simulink model "ScpAp_SpeedSupervision"  (R2025b)
settings: Solver=FixedStepDiscrete  StartTime=0.0  StopTime=10.0  FixedStep=0.01  RelTol=1e-3
model workspace (MAT data in the model file):
  K_Pred = Simulink.Parameter
  K_Pred.Value = 0.003
  K_Pred.Complexity = 'real'
  K_Pred.Dimensions = [1 1]
  K_Pred.DataType = 'auto'
  TH_Hystersis = Simulink.Parameter
  TH_Hystersis.Value = 3
  TH_Hystersis.Complexity = 'real'
  TH_Hystersis.Dimensions = [1 1]
  TH_Hystersis.DataType = 'auto'
  TH_Mon_Accel_Diff = Simulink.Parameter
  TH_Mon_Accel_Diff.Value = 2
  TH_Mon_Accel_Diff.Complexity = 'real'
  TH_Mon_Accel_Diff.Dimensions = [1 1]
  TH_Mon_Accel_Diff.DataType = 'auto'
  TH_Mon_Speed_Diff = Simulink.Parameter
  TH_Mon_Speed_Diff.Value = 2
  TH_Mon_Speed_Diff.Complexity = 'real'
  TH_Mon_Speed_Diff.Dimensions = [1 1]
  TH_Mon_Speed_Diff.DataType = 'auto'
  TH_Pred_Margin = Simulink.Parameter
  TH_Pred_Margin.Value = 2
  TH_Pred_Margin.Complexity = 'real'
  TH_Pred_Margin.Dimensions = [1 1]
  TH_Pred_Margin.DataType = 'auto'
  TH_Speed_Limit_Margin = Simulink.Parameter
  TH_Speed_Limit_Margin.Value = 3
  TH_Speed_Limit_Margin.Complexity = 'real'
  TH_Speed_Limit_Margin.Dimensions = [1 1]
  TH_Speed_Limit_Margin.DataType = 'auto'
  Torque_Decel_Limit = Simulink.Parameter
  Torque_Decel_Limit.Value = 500
  Torque_Decel_Limit.Complexity = 'real'
  Torque_Decel_Limit.Dimensions = [1 1]
  Torque_Decel_Limit.DataType = 'auto'
  Torque_PreLimit = Simulink.Parameter
  Torque_PreLimit.Value = 600
  Torque_PreLimit.Complexity = 'real'
  Torque_PreLimit.Dimensions = [1 1]
  Torque_PreLimit.DataType = 'auto'
undefined symbols (not defined in the file): SafetyMode_L2p_IDT, WhlSpd_Max
settings Model: DataDictionary=EgasPOC.sldd  Creator=IAST283  LastModifiedBy=IAST283
settings DataIOCC: SaveFormat=StructureWithTime
settings OptimizationCC: DefaultParameterBehavior=Inlined  EnhancedBackFolding=on  PassReuseOutputArgsAs=Individual arguments  ZeroExternalMemoryAtStartup=off  ZeroInternalMemoryAtStartup=off  OptimizeBlockOrder=speed  DifferentSizesBufferReuse=on  OptimizationCustomize=off  EfficientTunableParamExpr=on
settings DebuggingCC: ParameterTunabilityLossMsg=error
settings SFSimCC: MATLABDynamicMemAlloc=off
settings RTWCC: SystemTargetFile=autosar.tlc  GenCodeOnly=on  TemplateMakefile=ert_default_tmf  DataTypeReplacement=CDataTypesFixedWidth  Description=AUTOSAR
settings CodeAppCC: ForceParamTrailComments=on  IgnoreCustomStorageClasses=off  OperatorAnnotations=on  SimulinkDataObjDesc=on  SFDataObjDesc=on  InsertBlockDesc=on
settings STFCustomTargetCC: SystemTargetFile=autosar.tlc  TargetLangStandard=C99 (ISO)  MultiwordLength=256.0  ParMdlRefBuildCompliant=on  CompOptLevelCompliant=on  ConcurrentExecutionCompliant=off  IncludeMdlTerminateFcn=off  CombineOutputUpdateFcns=on  SuppressErrorStatus=on  ERTCustomFileBanners=on  SupportNonFinite=off  SupportComplex=off  SupportContinuousTime=off  SupportNonInlinedSFcns=off  RemoveResetFunc=on  MATLABClassNameForMDSCustomization=Simulink.SoftwareTarget.ERTCustomization  AutosarCompliant=on  GRTInterface=off  UseToolchainInfoCompliant=on  LookupTableObjectStructAxisOrder=2,1,3,4,...  LUTObjectStructOrderEvenSpacing=Size,Table,Breakpoints  AutosarMatrixIOAsArray=off  AutosarCompilerAbstraction=off  AutosarMaxShortNameLength=128.0  AutosarSchemaVersion=R20-11  DisableAUTOSARRoutinesHostLibrary=off
settings ERTTargetCC: ERTCustomFileTemplate=example_file_process.tlc  BooleanTrueId=TRUE  BooleanFalseId=FALSE  TargetLangStandard=C99 (ISO)  ConcurrentExecutionCompliant=off  IncludeMdlTerminateFcn=off  SuppressErrorStatus=on  SupportNonFinite=off  SupportComplex=off  ModelStepFunctionPrototypeControlCompliant=off  CPPClassGenCompliant=off  AutosarCompliant=on  LookupTableObjectStructAxisOrder=2,1,3,4,...  LUTObjectStructOrderEvenSpacing=Size,Table,Breakpoints

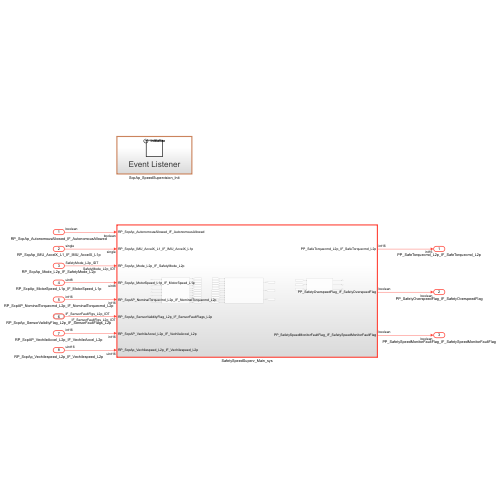
[thumbnail: Simulink's stored preview of the top-level diagram]
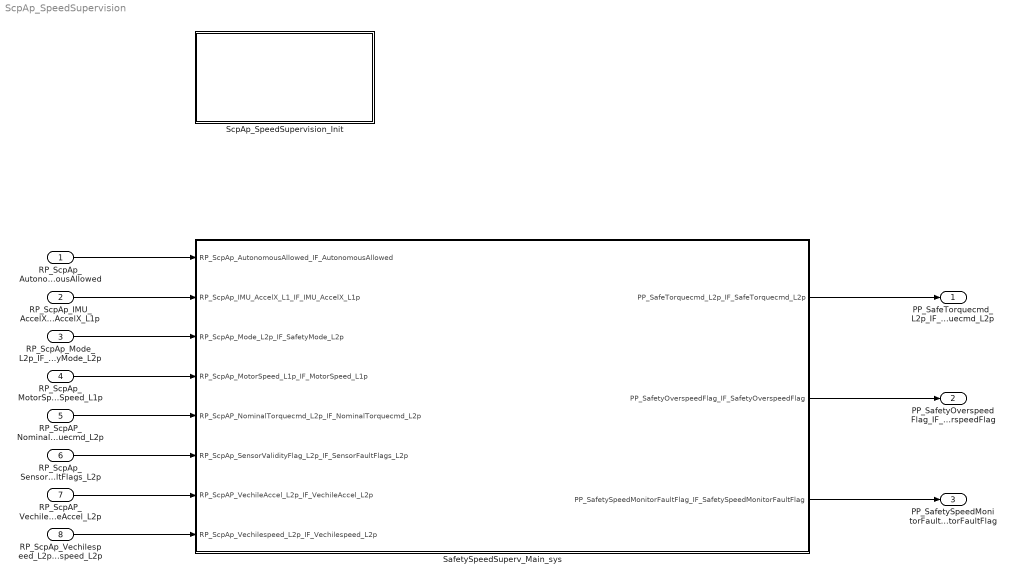
== system ScpAp_SpeedSupervision ==
  RP_ScpAp_AutonomousAllowed_IF_AutonomousAllowed : Inport  OutDataTypeStr=boolean  PortDimensions=1
  RP_ScpAp_IMU_AccelX_L1_IF_IMU_AccelX_L1p : Inport  Port=2  OutDataTypeStr=single  PortDimensions=1
  RP_ScpAp_Mode_L2p_IF_SafetyMode_L2p : Inport  Port=3  OutDataTypeStr=Enum: SafetyMode_L2p_IDT  PortDimensions=1
  RP_ScpAp_MotorSpeed_L1p_IF_MotorSpeed_L1p : Inport  Port=4  OutDataTypeStr=uint8  PortDimensions=1
  RP_ScpAP_NominalTorquecmd_L2p_IF_NominalTorquecmd_L2p : Inport  Port=5  OutDataTypeStr=int16  PortDimensions=1
  RP_ScpAp_SensorValidityFlag_L2p_IF_SensorFaultFlags_L2p : Inport  Port=6  OutDataTypeStr=Bus: IF_SensorFaultFlgs_L2p_IDT  PortDimensions=1  BusOutputAsStruct=on
  RP_ScpAP_VechileAccel_L2p_IF_VechileAccel_L2p : Inport  Port=7  OutDataTypeStr=int16  PortDimensions=1
  RP_ScpAp_Vechilespeed_L2p_IF_Vechilespeed_L2p : Inport  Port=8  OutDataTypeStr=uint16  PortDimensions=1
  SafetySpeedSuperv_Main_sys : Subsystem  TreatAsAtomicUnit=on  SystemSampleTime=0.01
  ScpAp_SpeedSupervision_Init : Subsystem
  PP_SafeTorquecmd_L2p_IF_SafeTorquecmd_L2p : Outport  OutDataTypeStr=int16  PortDimensions=1
  PP_SafetyOverspeedFlag_IF_SafetyOverspeedFlag : Outport  Port=2  OutDataTypeStr=boolean  PortDimensions=1
  PP_SafetySpeedMonitorFaultFlag_IF_SafetySpeedMonitorFaultFlag : Outport  Port=3  OutDataTypeStr=boolean  PortDimensions=1
  wires:
  RP_ScpAp_AutonomousAllowed_IF_AutonomousAllowed/1 -> SafetySpeedSuperv_Main_sys/1(RP_ScpAp_AutonomousAllowed_IF_AutonomousAllowed)
  RP_ScpAp_IMU_AccelX_L1_IF_IMU_AccelX_L1p/1 -> SafetySpeedSuperv_Main_sys/2(RP_ScpAp_IMU_AccelX_L1_IF_IMU_AccelX_L1p)
  RP_ScpAp_Mode_L2p_IF_SafetyMode_L2p/1 -> SafetySpeedSuperv_Main_sys/3(RP_ScpAp_Mode_L2p_IF_SafetyMode_L2p)
  RP_ScpAp_MotorSpeed_L1p_IF_MotorSpeed_L1p/1 -> SafetySpeedSuperv_Main_sys/4(RP_ScpAp_MotorSpeed_L1p_IF_MotorSpeed_L1p)
  RP_ScpAP_NominalTorquecmd_L2p_IF_NominalTorquecmd_L2p/1 -> SafetySpeedSuperv_Main_sys/5(RP_ScpAP_NominalTorquecmd_L2p_IF_NominalTorquecmd_L2p)
  RP_ScpAp_SensorValidityFlag_L2p_IF_SensorFaultFlags_L2p/1 -> SafetySpeedSuperv_Main_sys/6(RP_ScpAp_SensorValidityFlag_L2p_IF_SensorFaultFlags_L2p)
  RP_ScpAP_VechileAccel_L2p_IF_VechileAccel_L2p/1 -> SafetySpeedSuperv_Main_sys/7(RP_ScpAP_VechileAccel_L2p_IF_VechileAccel_L2p)
  RP_ScpAp_Vechilespeed_L2p_IF_Vechilespeed_L2p/1 -> SafetySpeedSuperv_Main_sys/8(RP_ScpAp_Vechilespeed_L2p_IF_Vechilespeed_L2p)
  SafetySpeedSuperv_Main_sys/1(PP_SafeTorquecmd_L2p_IF_SafeTorquecmd_L2p) -> PP_SafeTorquecmd_L2p_IF_SafeTorquecmd_L2p/1
  SafetySpeedSuperv_Main_sys/2(PP_SafetyOverspeedFlag_IF_SafetyOverspeedFlag) -> PP_SafetyOverspeedFlag_IF_SafetyOverspeedFlag/1
  SafetySpeedSuperv_Main_sys/3(PP_SafetySpeedMonitorFaultFlag_IF_SafetySpeedMonitorFaultFlag) -> PP_SafetySpeedMonitorFaultFlag_IF_SafetySpeedMonitorFaultFlag/1

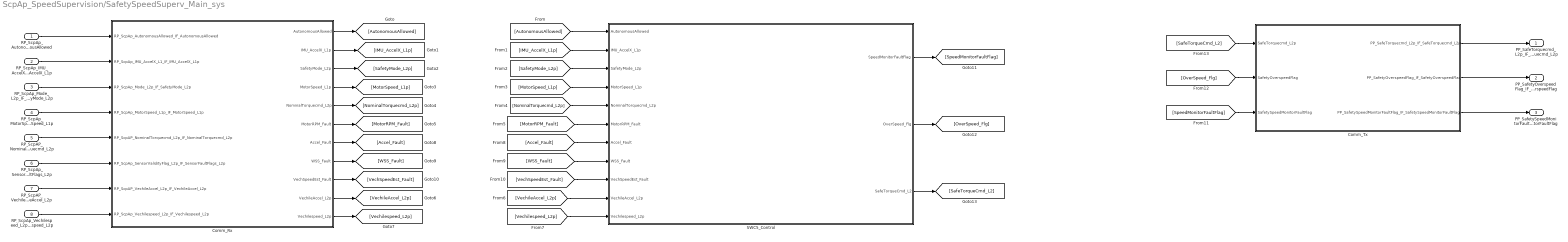
== system ScpAp_SpeedSupervision/SafetySpeedSuperv_Main_sys ==
  RP_ScpAp_AutonomousAllowed_IF_AutonomousAllowed : Inport
  RP_ScpAp_IMU_AccelX_L1_IF_IMU_AccelX_L1p : Inport  Port=2
  RP_ScpAp_Mode_L2p_IF_SafetyMode_L2p : Inport  Port=3
  RP_ScpAp_MotorSpeed_L1p_IF_MotorSpeed_L1p : Inport  Port=4
  RP_ScpAP_NominalTorquecmd_L2p_IF_NominalTorquecmd_L2p : Inport  Port=5
  RP_ScpAp_SensorValidityFlag_L2p_IF_SensorFaultFlags_L2p : Inport  Port=6
  RP_ScpAP_VechileAccel_L2p_IF_VechileAccel_L2p : Inport  Port=7
  RP_ScpAp_Vechilespeed_L2p_IF_Vechilespeed_L2p : Inport  Port=8
  Comm_Rx : Subsystem  TreatAsAtomicUnit=on
  Comm_Tx : Subsystem  TreatAsAtomicUnit=on
  SWC5_Control : Subsystem  TreatAsAtomicUnit=on
  PP_SafeTorquecmd_L2p_IF_SafeTorquecmd_L2p : Outport
  PP_SafetyOverspeedFlag_IF_SafetyOverspeedFlag : Outport  Port=2
  PP_SafetySpeedMonitorFaultFlag_IF_SafetySpeedMonitorFaultFlag : Outport  Port=3
  wires:
  RP_ScpAp_AutonomousAllowed_IF_AutonomousAllowed/1 -> Comm_Rx/1(RP_ScpAp_AutonomousAllowed_IF_AutonomousAllowed)
  RP_ScpAp_Vechilespeed_L2p_IF_Vechilespeed_L2p/1 -> Comm_Rx/8(RP_ScpAp_Vechilespeed_L2p_IF_Vechilespeed_L2p)
  RP_ScpAP_VechileAccel_L2p_IF_VechileAccel_L2p/1 -> Comm_Rx/7(RP_ScpAP_VechileAccel_L2p_IF_VechileAccel_L2p)
  RP_ScpAp_SensorValidityFlag_L2p_IF_SensorFaultFlags_L2p/1 -> Comm_Rx/6(RP_ScpAp_SensorValidityFlag_L2p_IF_SensorFaultFlags_L2p)
  RP_ScpAP_NominalTorquecmd_L2p_IF_NominalTorquecmd_L2p/1 -> Comm_Rx/5(RP_ScpAP_NominalTorquecmd_L2p_IF_NominalTorquecmd_L2p)
  RP_ScpAp_MotorSpeed_L1p_IF_MotorSpeed_L1p/1 -> Comm_Rx/4(RP_ScpAp_MotorSpeed_L1p_IF_MotorSpeed_L1p)
  RP_ScpAp_Mode_L2p_IF_SafetyMode_L2p/1 -> Comm_Rx/3(RP_ScpAp_Mode_L2p_IF_SafetyMode_L2p)
  RP_ScpAp_IMU_AccelX_L1_IF_IMU_AccelX_L1p/1 -> Comm_Rx/2(RP_ScpAp_IMU_AccelX_L1_IF_IMU_AccelX_L1p)
  Comm_Rx/1(AutonomousAllowed) -> [AutonomousAllowed]
  Comm_Rx/2(IMU_AccelX_L1p) -> [IMU_AccelX_L1p]
  Comm_Rx/3(SafetyMode_L2p) -> [SafetyMode_L2p]
  Comm_Rx/4(MotorSpeed_L1p) -> [MotorSpeed_L1p]
  Comm_Rx/5(NominalTorquecmd_L2p) -> [NominalTorquecmd_L2p]
  Comm_Rx/6(MotorRPM_Fault) -> [MotorRPM_Fault]
  Comm_Rx/10(VechileAccel_L2p) -> [VechileAccel_L2p]
  Comm_Rx/11(Vechilespeed_L2p) -> [Vechilespeed_L2p]
  Comm_Tx/1(PP_SafeTorquecmd_L2p_IF_SafeTorquecmd_L2p) -> PP_SafeTorquecmd_L2p_IF_SafeTorquecmd_L2p/1
  Comm_Tx/2(PP_SafetyOverspeedFlag_IF_SafetyOverspeedFlag) -> PP_SafetyOverspeedFlag_IF_SafetyOverspeedFlag/1
  Comm_Tx/3(PP_SafetySpeedMonitorFaultFlag_IF_SafetySpeedMonitorFaultFlag) -> PP_SafetySpeedMonitorFaultFlag_IF_SafetySpeedMonitorFaultFlag/1
  [AutonomousAllowed] -> SWC5_Control/1(AutonomousAllowed)
  [IMU_AccelX_L1p] -> SWC5_Control/2(IMU_AccelX_L1p)
  [SafetyMode_L2p] -> SWC5_Control/3(SafetyMode_L2p)
  [MotorSpeed_L1p] -> SWC5_Control/4(MotorSpeed_L1p)
  [NominalTorquecmd_L2p] -> SWC5_Control/5(NominalTorquecmd_L2p)
  [VechileAccel_L2p] -> SWC5_Control/10(VechileAccel_L2p)
  [Vechilespeed_L2p] -> SWC5_Control/11(Vechilespeed_L2p)
  Comm_Rx/8(WSS_Fault) -> [WSS_Fault]
  Comm_Rx/9(VechSpeedEst_Fault) -> [VechSpeedEst_Fault]
  [MotorRPM_Fault] -> SWC5_Control/6(MotorRPM_Fault)
  [Accel_Fault] -> SWC5_Control/7(Accel_Fault)
  [WSS_Fault] -> SWC5_Control/8(WSS_Fault)
  [VechSpeedEst_Fault] -> SWC5_Control/9(VechSpeedEst_Fault)
  Comm_Rx/7(Accel_Fault) -> [Accel_Fault]
  SWC5_Control/1(SpeedMonitorFaultFlag) -> [SpeedMonitorFaultFlag]
  SWC5_Control/2(OverSpeed_Flg) -> [OverSpeed_Flg]
  SWC5_Control/3(SafeTorqueCmd_L2) -> [SafeTorqueCmd_L2]
  [SpeedMonitorFaultFlag] -> Comm_Tx/3(SafetySpeedMonitorFaultFlag)
  [OverSpeed_Flg] -> Comm_Tx/2(SafetyOverspeedFlag)
  [SafeTorqueCmd_L2] -> Comm_Tx/1(SafeTorquecmd_L2p)

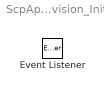
== system ScpAp_SpeedSupervision/ScpAp_SpeedSupervision_Init ==
  Event Listener : EventListener  EventName=reset

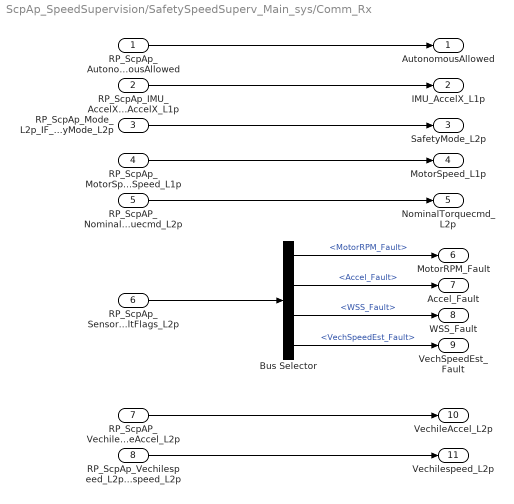
== system ScpAp_SpeedSupervision/SafetySpeedSuperv_Main_sys/Comm_Rx ==
  RP_ScpAp_AutonomousAllowed_IF_AutonomousAllowed : Inport
  RP_ScpAp_IMU_AccelX_L1_IF_IMU_AccelX_L1p : Inport  Port=2
  RP_ScpAp_Mode_L2p_IF_SafetyMode_L2p : Inport  Port=3
  RP_ScpAp_MotorSpeed_L1p_IF_MotorSpeed_L1p : Inport  Port=4
  RP_ScpAP_NominalTorquecmd_L2p_IF_NominalTorquecmd_L2p : Inport  Port=5
  RP_ScpAp_SensorValidityFlag_L2p_IF_SensorFaultFlags_L2p : Inport  Port=6
  RP_ScpAP_VechileAccel_L2p_IF_VechileAccel_L2p : Inport  Port=7
  RP_ScpAp_Vechilespeed_L2p_IF_Vechilespeed_L2p : Inport  Port=8
  Bus Selector : BusSelector  OutputSignals=MotorRPM_Fault,Accel_Fault,WSS_Fault,VechSpeedEst_Fault
  AutonomousAllowed : Outport
  IMU_AccelX_L1p : Outport  Port=2
  SafetyMode_L2p : Outport  Port=3
  MotorSpeed_L1p : Outport  Port=4
  NominalTorquecmd_L2p : Outport  Port=5
  MotorRPM_Fault : Outport  Port=6
  Accel_Fault : Outport  Port=7
  WSS_Fault : Outport  Port=8
  VechSpeedEst_Fault : Outport  Port=9
  VechileAccel_L2p : Outport  Port=10
  Vechilespeed_L2p : Outport  Port=11
  wires:
  RP_ScpAp_Vechilespeed_L2p_IF_Vechilespeed_L2p/1 -> Vechilespeed_L2p/1
  RP_ScpAP_NominalTorquecmd_L2p_IF_NominalTorquecmd_L2p/1 -> NominalTorquecmd_L2p/1
  RP_ScpAp_Mode_L2p_IF_SafetyMode_L2p/1 -> SafetyMode_L2p/1
  RP_ScpAp_MotorSpeed_L1p_IF_MotorSpeed_L1p/1 -> MotorSpeed_L1p/1
  RP_ScpAp_IMU_AccelX_L1_IF_IMU_AccelX_L1p/1 -> IMU_AccelX_L1p/1
  RP_ScpAP_VechileAccel_L2p_IF_VechileAccel_L2p/1 -> VechileAccel_L2p/1
  RP_ScpAp_SensorValidityFlag_L2p_IF_SensorFaultFlags_L2p/1 -> Bus Selector/1
  Bus Selector/1 -> MotorRPM_Fault/1  "<MotorRPM_Fault>"
  Bus Selector/2 -> Accel_Fault/1  "<Accel_Fault>"
  Bus Selector/3 -> WSS_Fault/1  "<WSS_Fault>"
  Bus Selector/4 -> VechSpeedEst_Fault/1  "<VechSpeedEst_Fault>"
  RP_ScpAp_AutonomousAllowed_IF_AutonomousAllowed/1 -> AutonomousAllowed/1

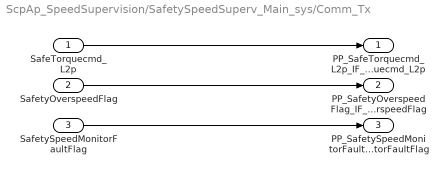
== system ScpAp_SpeedSupervision/SafetySpeedSuperv_Main_sys/Comm_Tx ==
  SafeTorquecmd_L2p : Inport
  SafetyOverspeedFlag : Inport  Port=2
  SafetySpeedMonitorFaultFlag : Inport  Port=3
  PP_SafeTorquecmd_L2p_IF_SafeTorquecmd_L2p : Outport
  PP_SafetyOverspeedFlag_IF_SafetyOverspeedFlag : Outport  Port=2
  PP_SafetySpeedMonitorFaultFlag_IF_SafetySpeedMonitorFaultFlag : Outport  Port=3
  wires:
  SafetyOverspeedFlag/1 -> PP_SafetyOverspeedFlag_IF_SafetyOverspeedFlag/1
  SafetySpeedMonitorFaultFlag/1 -> PP_SafetySpeedMonitorFaultFlag_IF_SafetySpeedMonitorFaultFlag/1
  SafeTorquecmd_L2p/1 -> PP_SafeTorquecmd_L2p_IF_SafeTorquecmd_L2p/1

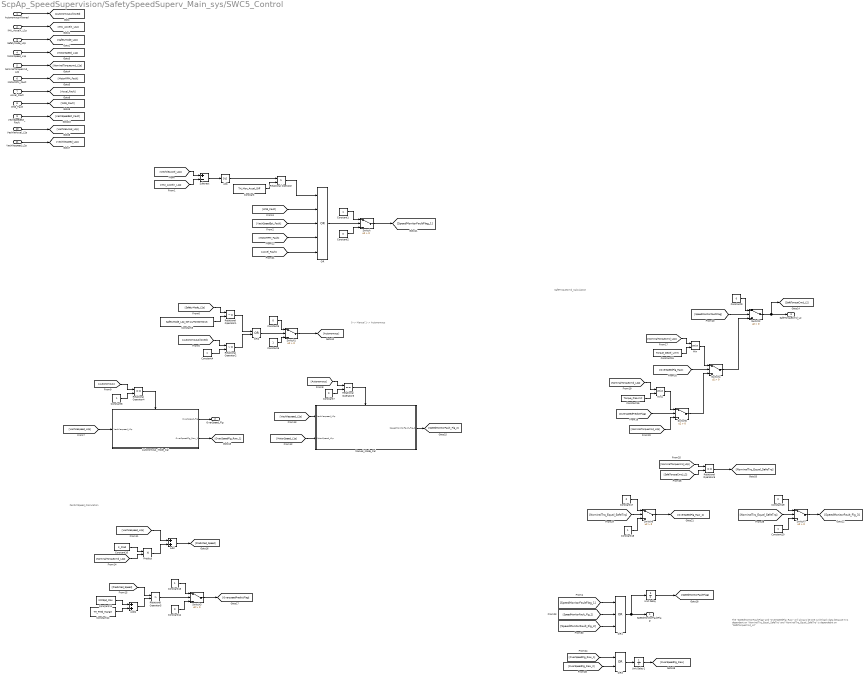
== system ScpAp_SpeedSupervision/SafetySpeedSuperv_Main_sys/SWC5_Control ==
  note: The "SpeedMonitorFaultFlag" and "OverSpeedFlg_Raw" will always be one cycle back data because it is dependent on "NominalTrq_Equal_SafeTrq" and "NominalTrq_Equal_SafeTrq" is dependednt on "SafeTorqueCmd_L2"
  note: SafeTroqueCmd_Calculation
  note: PerdictSpeed_Calculation
  note: 0 -> Manual
      | 1 -> Autonomous
  AutonomousAllowed : Inport
  IMU_AccelX_L1p : Inport  Port=2
  SafetyMode_L2p : Inport  Port=3
  MotorSpeed_L1p : Inport  Port=4
  NominalTorquecmd_L2p : Inport  Port=5
  MotorRPM_Fault : Inport  Port=6
  Accel_Fault : Inport  Port=7
  WSS_Fault : Inport  Port=8
  VechSpeedEst_Fault : Inport  Port=9
  VechileAccel_L2p : Inport  Port=10
  Vechilespeed_L2p : Inport  Port=11
  Abs : Abs  SaturateOnIntegerOverflow=off
  Add : Sum
  Add1 : Sum
  Autonomous_Mode_Cal : Subsystem
  Constant : Constant  Value=TH_Mon_Accel_Diff
  Constant{1,8,13,18,20} (5 alike) : Constant
  Constant10 : Constant  Value=K_Pred
  Constant11 : Constant  Value=WhlSpd_Max
  Constant12 : Constant  Value=TH_Pred_Margin
  Constant{2,7,14,17,19} (5 alike) : Constant  Value=0
  Constant15 : Constant  Value=Torque_Decel_Limit  OutDataTypeStr=int16
  Constant16 : Constant  Value=Torque_PreLimit  OutDataTypeStr=int16
  Constant3 : Constant  Value=SafetyMode_L2p_IDT.AUTONOMOUS
  Constant4 : Constant  OutDataTypeStr=boolean
  Constant5 : Constant  Value=0  OutDataTypeStr=boolean
  Constant6 : Constant  OutDataTypeStr=boolean
  Constant9 : Constant  Value=0  OutDataTypeStr=int16
  Manual_Mode_Cal : Subsystem
  Min : MinMax  Inputs=2  OutDataTypeStr=int16
  Min1 : MinMax  Inputs=2  OutDataTypeStr=int16
  OR : Logic  Operator=OR  Inputs=5  AllPortsSameDT=off  OutDataTypeStr=boolean
  OR1 : Logic  Operator=OR  Inputs=3  AllPortsSameDT=off  OutDataTypeStr=boolean
  OR2 : Logic  Operator=OR  AllPortsSameDT=off  OutDataTypeStr=boolean
  OR3 : Logic  Operator=OR  AllPortsSameDT=off  OutDataTypeStr=boolean
  Product : Product
  Relational Operator : RelationalOperator  Operator=>  OutDataTypeStr=boolean  RndMeth=Simplest  InputSameDT=off
  Relational Operator1 : RelationalOperator  Operator=~=  OutDataTypeStr=boolean  RndMeth=Simplest  InputSameDT=off
  Relational Operator2 : RelationalOperator  Operator=~=  OutDataTypeStr=boolean  RndMeth=Simplest  InputSameDT=off
  Relational Operator3 : RelationalOperator  Operator===  OutDataTypeStr=boolean  RndMeth=Simplest  InputSameDT=off
  Relational Operator4 : RelationalOperator  Operator===  OutDataTypeStr=boolean  RndMeth=Simplest  InputSameDT=off
  Relational Operator5 : RelationalOperator  Operator=>  OutDataTypeStr=boolean  RndMeth=Simplest  InputSameDT=off
  Relational Operator6 : RelationalOperator  Operator===  OutDataTypeStr=boolean  RndMeth=Simplest  InputSameDT=off
  Subtract : Sum  Inputs=+-
  Switch{,1..7} (8 alike) : Switch  Criteria=u2 > Threshold  SaturateOnIntegerOverflow=off  InputSameDT=off
  Unit Delay : UnitDelay  SampleTime=-1  HasFrameUpgradeWarning=on
  Unit Delay1 : UnitDelay  SampleTime=-1  HasFrameUpgradeWarning=on
  SpeedMonitorFaultFlag : Outport
  OverSpeed_Flg : Outport  Port=2
  SafeTorqueCmd_L2 : Outport  Port=3
  wires:
  AutonomousAllowed/1 -> [AutonomousAllowed]
  IMU_AccelX_L1p/1 -> [IMU_AccelX_L1p]
  SafetyMode_L2p/1 -> [SafetyMode_L2p]
  MotorSpeed_L1p/1 -> [MotorSpeed_L1p]
  MotorRPM_Fault/1 -> [MotorRPM_Fault]
  NominalTorquecmd_L2p/1 -> [NominalTorquecmd_L2p]
  VechileAccel_L2p/1 -> [VechileAccel_L2p]
  Vechilespeed_L2p/1 -> [Vechilespeed_L2p]
  WSS_Fault/1 -> [WSS_Fault]
  Accel_Fault/1 -> [Accel_Fault]
  VechSpeedEst_Fault/1 -> [VechSpeedEst_Fault]
  [VechileAccel_L2p] -> Subtract/1
  [IMU_AccelX_L1p] -> Subtract/2
  Subtract/1 -> Abs/1
  Abs/1 -> Relational Operator/1
  Constant/1 -> Relational Operator/2
  Relational Operator/1 -> OR/1
  [VechSpeedEst_Fault] -> OR/3
  [WSS_Fault] -> OR/2
  OR/1 -> Switch/2
  Switch/1 -> [SpeedMonitorFaultFlag_1]
  Constant1/1 -> Switch/1
  Constant2/1 -> Switch/3
  [SpeedMonitorFaultFlag_1] -> OR1/1
  [SafetyMode_L2p] -> Relational Operator1/1
  Constant3/1 -> Relational Operator1/2
  Relational Operator1/1 -> OR2/1
  [AutonomousAllowed] -> Relational Operator2/1
  Constant4/1 -> Relational Operator2/2
  Relational Operator2/1 -> OR2/2
  OR2/1 -> Switch1/2
  [Vechilespeed_L2p] -> Autonomous_Mode_Cal/1(Vechilespeed_L2p)
  Autonomous_Mode_Cal/1(OverSpeed_Flg) -> OverSpeed_Flg/1
  [Vechilespeed_L2p] -> Manual_Mode_Cal/1(Vechilespeed_L2p)
  [MotorSpeed_L1p] -> Manual_Mode_Cal/2(MotorSpeed_L1p)
  Manual_Mode_Cal/1(SpeedMonitorFault_Flg_2) -> [SpeedMonitorFault_Flg_2]
  Constant5/1 -> Switch1/1
  Constant6/1 -> Switch1/3
  [Autonomous] -> Relational Operator3/1
  Constant7/1 -> Relational Operator3/2
  Relational Operator3/1 -> Manual_Mode_Cal/Enable
  [Autonomous] -> Relational Operator4/1
  Constant8/1 -> Relational Operator4/2
  Relational Operator4/1 -> Autonomous_Mode_Cal/Enable
  Autonomous_Mode_Cal/2(OverSpeedFlg_Raw_1) -> [OverSpeedFlg_Raw_1]
  [SpeedMonitorFaultFlag] -> Switch2/2
  Switch2/1 -> [SafeTorqueCmd_L2], SafeTorqueCmd_L2/1
  Constant9/1 -> Switch2/1
  Constant10/1 -> Product/1
  [NominalTorquecmd_L2p] -> Product/2
  Product/1 -> Add/2
  [Vechilespeed_L2p] -> Add/1
  Add/1 -> [Predicted_Speed]
  [Predicted_Speed] -> Relational Operator5/1
  Add1/1 -> Relational Operator5/2
  Constant11/1 -> Add1/1
  Constant12/1 -> Add1/2
  Relational Operator5/1 -> Switch3/2
  Switch3/1 -> [OverspeedPredictFlag]
  Constant13/1 -> Switch3/1
  Constant14/1 -> Switch3/3
  [OverSpeedFlg_Raw] -> Switch4/2
  [NominalTorquecmd_L2p] -> Min/1
  Constant15/1 -> Min/2
  Min/1 -> Switch4/1
  Switch4/1 -> Switch2/3
  [OverspeedPredictFlag] -> Switch5/2
  Min1/1 -> Switch5/1
  [NominalTorquecmd_L2p] -> Min1/1
  Constant16/1 -> Min1/2
  Switch5/1 -> Switch4/3
  [NominalTorquecmd_L2p] -> Switch5/3
  [MotorRPM_Fault] -> OR/4
  [Accel_Fault] -> OR/5
  [SpeedMonitorFault_Flg_2] -> OR1/2
  [OverSpeedFlg_Raw_1] -> OR3/1
  OR3/1 -> Unit Delay1/1
  [NominalTorquecmd_L2p] -> Relational Operator6/1
  [SafeTorqueCmd_L2] -> Relational Operator6/2
  Relational Operator6/1 -> [NominalTrq_Equal_SafeTrq]
  [NominalTrq_Equal_SafeTrq] -> Switch6/2
  Switch6/1 -> [OverSpeedFlg_Raw_2]
  Constant17/1 -> Switch6/1
  Constant18/1 -> Switch6/3
  [OverSpeedFlg_Raw_2] -> OR3/2
  [NominalTrq_Equal_SafeTrq] -> Switch7/2
  Switch7/1 -> [SpeedMonitorFault_Flg_3]
  Constant20/1 -> Switch7/3
  Constant19/1 -> Switch7/1
  [SpeedMonitorFault_Flg_3] -> OR1/3
  OR1/1 -> Unit Delay/1, SpeedMonitorFaultFlag/1
  Switch1/1 -> [Autonomous]
  Unit Delay/1 -> [SpeedMonitorFaultFlag]
  Unit Delay1/1 -> [OverSpeedFlg_Raw]

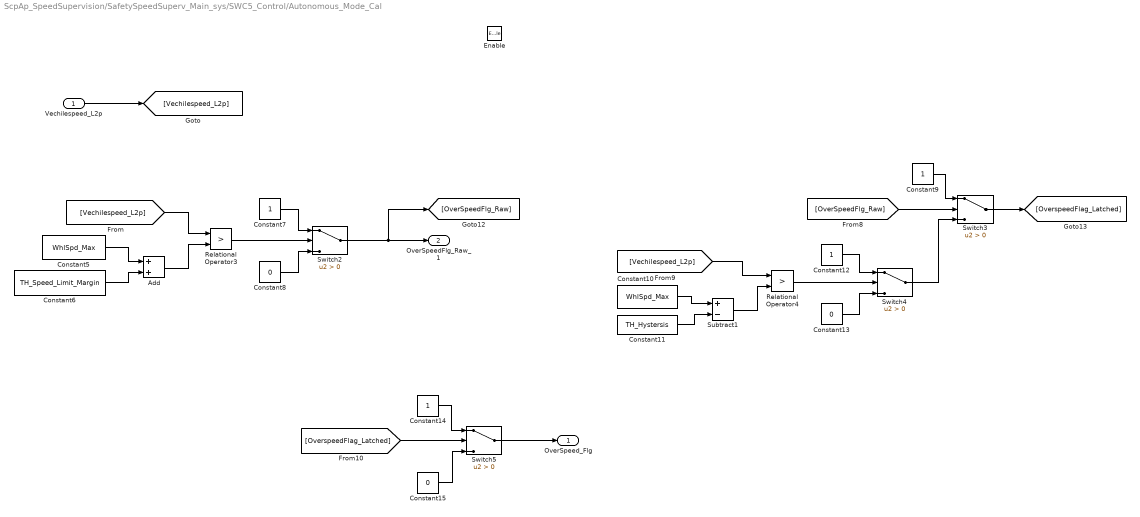
== system ScpAp_SpeedSupervision/SafetySpeedSuperv_Main_sys/SWC5_Control/Autonomous_Mode_Cal ==
  Vechilespeed_L2p : Inport
  Enable : EnablePort
  Add : Sum
  Constant10 : Constant  Value=WhlSpd_Max
  Constant11 : Constant  Value=TH_Hystersis
  Constant{7,9,12,14} (4 alike) : Constant  OutDataTypeStr=boolean
  Constant13 : Constant  Value=0  OutDataTypeStr=boolean
  Constant15 : Constant  Value=0  OutDataTypeStr=boolean
  Constant5 : Constant  Value=WhlSpd_Max
  Constant6 : Constant  Value=TH_Speed_Limit_Margin
  Constant8 : Constant  Value=0  OutDataTypeStr=boolean
  Relational Operator3 : RelationalOperator  Operator=>  OutDataTypeStr=boolean  RndMeth=Simplest  InputSameDT=off
  Relational Operator4 : RelationalOperator  Operator=>  OutDataTypeStr=boolean  RndMeth=Simplest  InputSameDT=off
  Subtract1 : Sum  Inputs=+-
  Switch{2..5} (4 alike) : Switch  Criteria=u2 > Threshold  SaturateOnIntegerOverflow=off  InputSameDT=off
  OverSpeed_Flg : Outport
  OverSpeedFlg_Raw_1 : Outport  Port=2
  wires:
  Switch2/1 -> OverSpeedFlg_Raw_1/1, [OverSpeedFlg_Raw]
  Constant7/1 -> Switch2/1
  Constant12/1 -> Switch4/1
  Relational Operator4/1 -> Switch4/2
  Constant10/1 -> Subtract1/1
  Switch4/1 -> Switch3/3
  Constant8/1 -> Switch2/3
  [OverSpeedFlg_Raw] -> Switch3/2
  Relational Operator3/1 -> Switch2/2
  Constant6/1 -> Add/2
  Constant15/1 -> Switch5/3
  Subtract1/1 -> Relational Operator4/2
  Constant13/1 -> Switch4/3
  Constant9/1 -> Switch3/1
  Add/1 -> Relational Operator3/2
  Switch3/1 -> [OverspeedFlag_Latched]
  [OverspeedFlag_Latched] -> Switch5/2
  Constant11/1 -> Subtract1/2
  Constant14/1 -> Switch5/1
  Constant5/1 -> Add/1
  [Vechilespeed_L2p] -> Relational Operator4/1
  Switch5/1 -> OverSpeed_Flg/1
  Vechilespeed_L2p/1 -> [Vechilespeed_L2p]
  [Vechilespeed_L2p] -> Relational Operator3/1

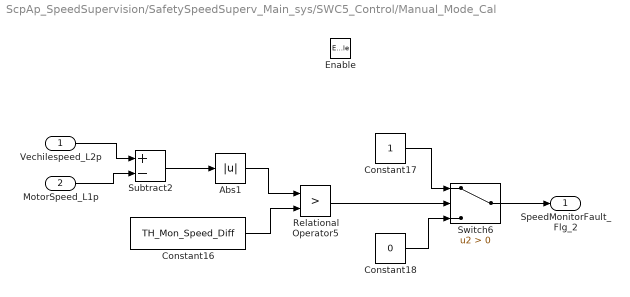
== system ScpAp_SpeedSupervision/SafetySpeedSuperv_Main_sys/SWC5_Control/Manual_Mode_Cal ==
  Vechilespeed_L2p : Inport
  MotorSpeed_L1p : Inport  Port=2
  Enable : EnablePort
  Abs1 : Abs  SaturateOnIntegerOverflow=off
  Constant16 : Constant  Value=TH_Mon_Speed_Diff
  Constant17 : Constant
  Constant18 : Constant  Value=0
  Relational Operator5 : RelationalOperator  Operator=>  OutDataTypeStr=boolean  RndMeth=Simplest  InputSameDT=off
  Subtract2 : Sum  Inputs=+-
  Switch6 : Switch  Criteria=u2 > Threshold  SaturateOnIntegerOverflow=off  InputSameDT=off
  SpeedMonitorFault_Flg_2 : Outport
  wires:
  Constant17/1 -> Switch6/1
  Subtract2/1 -> Abs1/1
  Relational Operator5/1 -> Switch6/2
  Abs1/1 -> Relational Operator5/1
  MotorSpeed_L1p/1 -> Subtract2/2
  Switch6/1 -> SpeedMonitorFault_Flg_2/1
  Constant18/1 -> Switch6/3
  Constant16/1 -> Relational Operator5/2
  Vechilespeed_L2p/1 -> Subtract2/1
